simulink model "p4"  (R2018a)
settings: Solver=VariableStepAuto  StartTime=0.0  StopTime=1  MaxStep=1e-3  RelTol=1e-3
values from neighbouring files (symbols this model uses):
  h3 = 2*tf([1 5],5)*tf(20,[1 20])*tf(50,[1 50])*tf([1 150],150)    [ef.m]
  h4 = 2*tf([1 20],20)*tf(5,[1 5])*tf(100,[1 100])*tf([1 50],50)    [ef.m]
  h5 = 2*tf([1 10],10)*tf(5,[1 5])*tf([1 20],20)*tf(50,[1 50])    [ef.m]
settings Model: Creator=carma  LastModifiedBy=carma

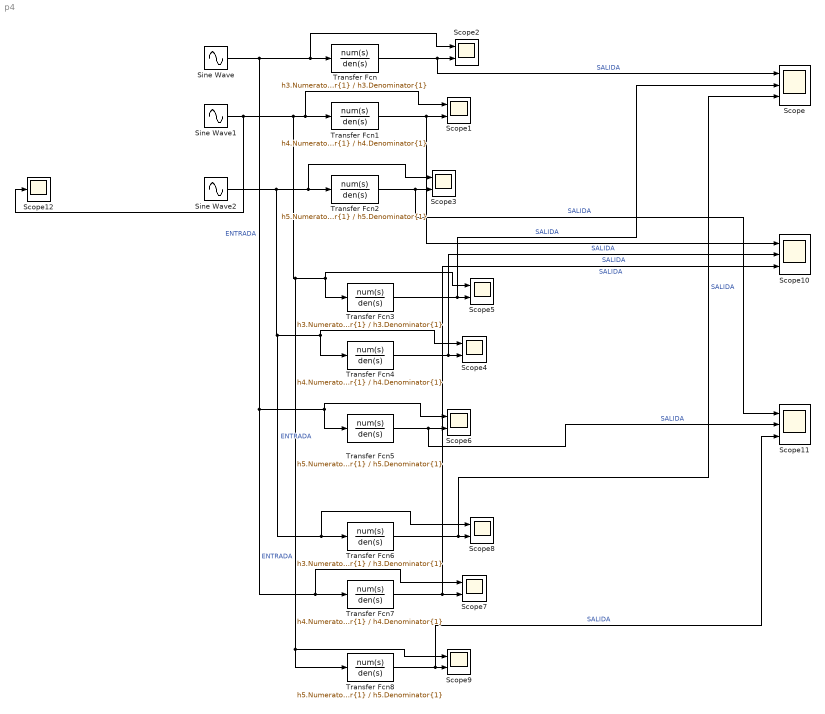
== system p4 ==
  Scope : Scope  NumInputPorts=3
  Scope{1..9} (9 alike) : Scope  NumInputPorts=2
  Scope10 : Scope  NumInputPorts=3
  Scope11 : Scope  NumInputPorts=3
  Scope12 : Scope
  Sine Wave : Sin  Frequency=34.7  SampleTime=0
  Sine Wave1 : Sin  Frequency=44.2  SampleTime=0
  Sine Wave2 : Sin  Frequency=12  SampleTime=0
  Transfer Fcn : TransferFcn  Numerator=h3.Numerator{1}  Denominator=h3.Denominator{1}
  Transfer Fcn1 : TransferFcn  Numerator=h4.Numerator{1}  Denominator=h4.Denominator{1}
  Transfer Fcn2 : TransferFcn  Numerator=h5.Numerator{1}  Denominator=h5.Denominator{1}
  Transfer Fcn3 : TransferFcn  Numerator=h3.Numerator{1}  Denominator=h3.Denominator{1}
  Transfer Fcn4 : TransferFcn  Numerator=h4.Numerator{1}  Denominator=h4.Denominator{1}
  Transfer Fcn5 : TransferFcn  Numerator=h5.Numerator{1}  Denominator=h5.Denominator{1}
  Transfer Fcn6 : TransferFcn  Numerator=h3.Numerator{1}  Denominator=h3.Denominator{1}
  Transfer Fcn7 : TransferFcn  Numerator=h4.Numerator{1}  Denominator=h4.Denominator{1}
  Transfer Fcn8 : TransferFcn  Numerator=h5.Numerator{1}  Denominator=h5.Denominator{1}
  wires:
  Transfer Fcn/1 -> Scope/1, Scope2/2  "SALIDA"
  Transfer Fcn2/1 -> Scope11/1, Scope3/2  "SALIDA"
  Transfer Fcn1/1 -> Scope10/1, Scope1/2  "SALIDA"
  Transfer Fcn5/1 -> Scope11/2, Scope6/2  "SALIDA"
  Transfer Fcn4/1 -> Scope10/2, Scope4/2  "SALIDA"
  Transfer Fcn3/1 -> Scope/2, Scope5/2  "SALIDA"
  Transfer Fcn6/1 -> Scope/3, Scope8/2  "SALIDA"
  Sine Wave1/1 -> Scope12/1, Transfer Fcn8/1, Scope9/1, Transfer Fcn3/1, Scope5/1, Scope1/1, Transfer Fcn1/1  "ENTRADA"
  Sine Wave2/1 -> Scope8/1, Transfer Fcn6/1, Transfer Fcn4/1, Scope4/1, Scope3/1, Transfer Fcn2/1  "ENTRADA"
  Transfer Fcn7/1 -> Scope10/3, Scope7/2  "SALIDA"
  Sine Wave/1 -> Scope7/1, Transfer Fcn7/1, Transfer Fcn5/1, Scope6/1, Scope2/1, Transfer Fcn/1  "ENTRADA"
  Transfer Fcn8/1 -> Scope11/3, Scope9/2  "SALIDA"
